simulink model "SimulationBlockDiagram"  (R2019b)
settings: Solver=VariableStepAuto  StartTime=0.0  StopTime=10.0  RelTol=1e-3
libraries: mobileRoboticsLib x3, simulink x2
settings Model: Creator=Douglas.C  LastModifiedBy=Douglas.C

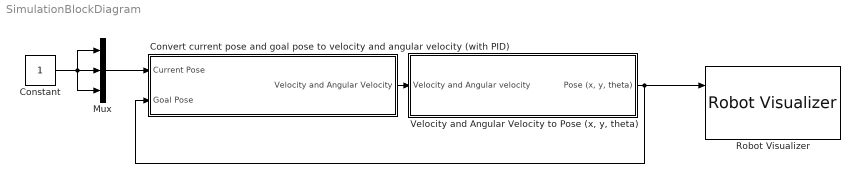
== system SimulationBlockDiagram ==
  Constant : Constant
  Convert current pose and goal pose to velocity and angular velocity (with PID) : Subsystem
  Mux : Mux  Inputs=3
  Robot Visualizer : mobileRoboticsLib/Environments/Robot Visualizer  robotRadius=0  showTrajectory=on  hasWaypoints=off  hasLidar=off  sensorOffset=[ 0, 0 ]  scanAngles=[ -pi/4, 0, pi/4 ]  hasObjDetector=on  objDetectorOffset=[ 0, 0 ]  objDetectorAngle=0  objDetectorFOV=pi/4  objDetectorMaxRange=5  objectColors=[ 1, 0, 0; 0, 1, 0; 0, 0, 1 ]  objectMarkers=s
  "Velocity and Angular Velocity to Pose (x, y, theta)" : Subsystem
  wires:
  Convert current pose and goal pose to velocity and angular velocity (with PID)/1(Velocity and Angular Velocity) -> "Velocity and Angular Velocity to Pose (x, y, theta)"/1(Velocity and Angular velocity)
  "Velocity and Angular Velocity to Pose (x, y, theta)"/1("Pose (x, y, theta)") -> Robot Visualizer/1, Convert current pose and goal pose to velocity and angular velocity (with PID)/2(Goal Pose)
  Mux/1 -> Convert current pose and goal pose to velocity and angular velocity (with PID)/1(Current Pose)
  Constant/1 -> Mux/1, Mux/3, Mux/2

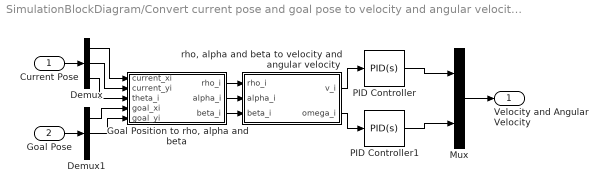
== system SimulationBlockDiagram/Convert current pose and goal pose to velocity and angular velocity (with PID) ==
  Current Pose : Inport
  Goal Pose : Inport  Port=2
  Demux : Demux  Outputs=3
  Demux1 : Demux  Outputs=3
  "Goal Position to rho, alpha and beta" : MATLAB Function  TreatAsAtomicUnit=on
  Mux : Mux  Inputs=2
  PID Controller : simulink/Continuous/PID Controller  Controller=PID  Form=Parallel  TimeDomain=Continuous-time  SampleTime=-1  IntegratorMethod=Forward Euler  FilterMethod=Forward Euler  ControllerParametersSource=internal  P=1  I=1  D=0  UseFilter=on  N=100  TunerSelectOption=Transfer Function Based (PID Tuner App)  InitialConditionSource=internal  InitialConditionForIntegrator=0  InitialConditionForFilter=0  DifferentiatorICPrevScaledInput=0  ExternalReset=none  TrackingMode=off  Kt=1  LimitOutput=off  UpperSaturationLimit=inf  LowerSaturationLimit=-inf  LinearizeAsGain=on  AntiWindupMode=none  Kb=1  POutMin=[]  POutMax=[]  IOutMin=[]  IOutMax=[]  DOutMin=[]  DOutMax=[]  NOutMin=[]  NOutMax=[]  SumOutMin=[]  SumOutMax=[]  SaturationOutMin=[]  SaturationOutMax=[]  PParamMin=[]  PParamMax=[]  IParamMin=[]  IParamMax=[]  DParamMin=[]  DParamMax=[]  NParamMin=[]  NParamMax=[]  KbParamMin=[]  KbParamMax=[]  KtParamMin=[]  KtParamMax=[]  KbOutMin=[]  KbOutMax=[]  KtOutMin=[]  KtOutMax=[]  IntegratorOutMin=[]  IntegratorOutMax=[]  FilterOutMin=[]  FilterOutMax=[]  SumI1OutMin=[]  SumI1OutMax=[]  SumI2OutMin=[]  SumI2OutMax=[]  SumI3OutMin=[]  SumI3OutMax=[]  SumI4OutMin=[]  SumI4OutMax=[]  SumDOutMin=[]  SumDOutMax=[]  DifferentiatorOutMin=[]  DifferentiatorOutMax=[]  FilterDiffOutCoefMin=[]  FilterDiffOutCoefMax=[]  ReciprocalOutMin=[]  ReciprocalOutMax=[]  SumDenOutMin=[]  SumDenOutMax=[]  SumNumOutMin=[]  SumNumOutMax=[]  DivideOutMin=[]  DivideOutMax=[]  IntegratorContinuousStateAttributes=''  IntegratorStateMustResolveToSignalObject=off  IntegratorRTWStateStorageClass=Auto  FilterContinuousStateAttributes=''  FilterStateMustResolveToSignalObject=off  FilterRTWStateStorageClass=Auto  ParallelPVariant=InternalParameters  IdealPVariant=Disabled  IVariant=InternalParameters  DVariant=InternalParameters  IntegratorVariant=Continuous  SatVariant=Disabled  AWVariant=Passthrough  PCopyVariant=Disabled  TRVariant=Disabled  FdbkBlocksVariant=Forward  IdealPFdbkVariant=Disabled  SatFdbkVariant=Disabled  DerivativeFilterVariant=ContFilter  NVariant=InternalParameters  NCopyVariant=Disabled  FilterICVariant=InternalICsFilter  IntegratorICVariant=InternalICs  ExternalResetVariant=Disabled  TRSumVariant=Passthrough  SumFdbkVariant=Disabled  SumVariant=Sum_PID
  PID Controller1 : simulink/Continuous/PID Controller  Controller=PID  Form=Parallel  TimeDomain=Continuous-time  SampleTime=-1  IntegratorMethod=Forward Euler  FilterMethod=Forward Euler  ControllerParametersSource=internal  P=1  I=1  D=0  UseFilter=on  N=100  TunerSelectOption=Transfer Function Based (PID Tuner App)  InitialConditionSource=internal  InitialConditionForIntegrator=0  InitialConditionForFilter=0  DifferentiatorICPrevScaledInput=0  ExternalReset=none  TrackingMode=off  Kt=1  LimitOutput=off  UpperSaturationLimit=inf  LowerSaturationLimit=-inf  LinearizeAsGain=on  AntiWindupMode=none  Kb=1  POutMin=[]  POutMax=[]  IOutMin=[]  IOutMax=[]  DOutMin=[]  DOutMax=[]  NOutMin=[]  NOutMax=[]  SumOutMin=[]  SumOutMax=[]  SaturationOutMin=[]  SaturationOutMax=[]  PParamMin=[]  PParamMax=[]  IParamMin=[]  IParamMax=[]  DParamMin=[]  DParamMax=[]  NParamMin=[]  NParamMax=[]  KbParamMin=[]  KbParamMax=[]  KtParamMin=[]  KtParamMax=[]  KbOutMin=[]  KbOutMax=[]  KtOutMin=[]  KtOutMax=[]  IntegratorOutMin=[]  IntegratorOutMax=[]  FilterOutMin=[]  FilterOutMax=[]  SumI1OutMin=[]  SumI1OutMax=[]  SumI2OutMin=[]  SumI2OutMax=[]  SumI3OutMin=[]  SumI3OutMax=[]  SumI4OutMin=[]  SumI4OutMax=[]  SumDOutMin=[]  SumDOutMax=[]  DifferentiatorOutMin=[]  DifferentiatorOutMax=[]  FilterDiffOutCoefMin=[]  FilterDiffOutCoefMax=[]  ReciprocalOutMin=[]  ReciprocalOutMax=[]  SumDenOutMin=[]  SumDenOutMax=[]  SumNumOutMin=[]  SumNumOutMax=[]  DivideOutMin=[]  DivideOutMax=[]  IntegratorContinuousStateAttributes=''  IntegratorStateMustResolveToSignalObject=off  IntegratorRTWStateStorageClass=Auto  FilterContinuousStateAttributes=''  FilterStateMustResolveToSignalObject=off  FilterRTWStateStorageClass=Auto  ParallelPVariant=InternalParameters  IdealPVariant=Disabled  IVariant=InternalParameters  DVariant=InternalParameters  IntegratorVariant=Continuous  SatVariant=Disabled  AWVariant=Passthrough  PCopyVariant=Disabled  TRVariant=Disabled  FdbkBlocksVariant=Forward  IdealPFdbkVariant=Disabled  SatFdbkVariant=Disabled  DerivativeFilterVariant=ContFilter  NVariant=InternalParameters  NCopyVariant=Disabled  FilterICVariant=InternalICsFilter  IntegratorICVariant=InternalICs  ExternalResetVariant=Disabled  TRSumVariant=Passthrough  SumFdbkVariant=Disabled  SumVariant=Sum_PID
  "rho, alpha and beta to velocity and angular velocity" : MATLAB Function  TreatAsAtomicUnit=on
  Velocity and Angular Velocity : Outport
  wires:
  Demux1/1 -> "Goal Position to rho, alpha and beta"/4(goal_xi)
  Goal Pose/1 -> Demux1/1
  PID Controller/1 -> Mux/1
  "rho, alpha and beta to velocity and angular velocity"/1(v_i) -> PID Controller/1
  Demux/2 -> "Goal Position to rho, alpha and beta"/2(current_yi)
  Demux1/2 -> "Goal Position to rho, alpha and beta"/5(goal_yi)
  "Goal Position to rho, alpha and beta"/2(alpha_i) -> "rho, alpha and beta to velocity and angular velocity"/2(alpha_i)
  "rho, alpha and beta to velocity and angular velocity"/2(omega_i) -> PID Controller1/1
  Demux/3 -> "Goal Position to rho, alpha and beta"/3(theta_i)
  Demux/1 -> "Goal Position to rho, alpha and beta"/1(current_xi)
  "Goal Position to rho, alpha and beta"/1(rho_i) -> "rho, alpha and beta to velocity and angular velocity"/1(rho_i)
  "Goal Position to rho, alpha and beta"/3(beta_i) -> "rho, alpha and beta to velocity and angular velocity"/3(beta_i)
  PID Controller1/1 -> Mux/2
  Current Pose/1 -> Demux/1
  Mux/1 -> Velocity and Angular Velocity/1

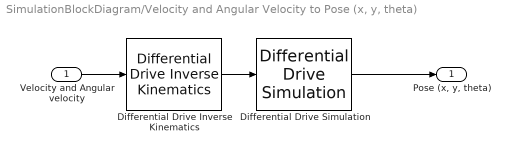
== system SimulationBlockDiagram/Velocity and Angular Velocity to Pose (x, y, theta) ==
  Velocity and Angular velocity : Inport
  Differential Drive Inverse Kinematics : mobileRoboticsLib/Kinematic Models/Differential Drive/Differential Drive Inverse Kinematics  wheelRadius=0.1  wheelBase=0.5
      settings: SourceProductName=Mobile Robotics Simulation Toolbox
  Differential Drive Simulation : mobileRoboticsLib/Kinematic Models/Differential Drive/Differential Drive Simulation  wheelRadius=0.1  wheelBase=0.5  initX=0  initY=0  initAngle=0  Ts=0.05
      settings: SourceProductName=Mobile Robotics Simulation Toolbox
  "Pose (x, y, theta)" : Outport
  wires:
  Differential Drive Simulation/1 -> "Pose (x, y, theta)"/1
  Differential Drive Inverse Kinematics/1 -> Differential Drive Simulation/1
  Velocity and Angular velocity/1 -> Differential Drive Inverse Kinematics/1

== matlab function SimulationBlockDiagram/Convert current pose and goal pose to velocity and angular velocity (with PID)/Goal Position to rho, alpha and beta ==
  data: current_xi input; rho_i output; current_yi input; alpha_i output; theta_i input; goal_xi input; goal_yi input; beta_i output
% **Description:
% This function convert the current pose and goal pose information to rho,
% alpha and beta for each robot agent
%
% **Variables Description:
%   Input:
%       current_xi: x-coordinate of current pose
%       current_yi: y-coordinate of current pose
%       theta_i:    Orientation (angle) of current pose
%
%       goal_xi:    x-coordinate of goal pose
%       goal_yi:    y-coordinate of goal pose
%
%   Output:
%       rho_i:      Distance between the Start pose and Goal pose
%       alpha_i:    Starting orientation (angle)
%       beta_i:     Goal orientation (angle)

function [rho_i, alpha_i, beta_i] = fcn(current_xi, current_yi, theta_i, goal_xi, goal_yi)
% Initialize:
rho_i    = 0.0;
alpha_i  = 0.0;
beta_i   = 0.0;

% Convert Parameters:
delta_xi = goal_xi - current_xi;
delta_yi = goal_yi - current_yi;

% Output:
rho_i    = sqrt(square(delta_xi) + square(delta_yi));
alpha_i  = atan(delta_yi/delta_xi) - theta_i;
beta_i   = - theta_i - alpha_i;

== matlab function SimulationBlockDiagram/Convert current pose and goal pose to velocity and angular velocity (with PID)/rho, alpha and beta to velocity and angular velocity ==
  data: rho_i input; v_i output; alpha_i input; omega_i output; beta_i input
% **Description:
% This function convert the information of the start pose and goal pose
% to velocity and angular velocity.
%
% **Variables Description:
%   Input:
%       rho_i:      Distance between the Start pose and Goal pose
%       alpha_i:    Starting orientation (angle)
%       beta_i:     Goal orientation (angle)
%
%   Tunning Parameters:
%       K_rho:      > 0
%       K_alpha:    > K_rho
%       K_beta:     < 0
%
%   Output:
%       v_i:        Linear velocity of robot agent i
%       omega_i:    Angular velocity of robot agent i

function [v_i, omega_i] = fcn(rho_i, alpha_i, beta_i)

% Tunning Parameters:
K_rho   = 5;
K_alpha = 10;
K_beta  = -0.1;

% Output
v_i     = K_rho*rho_i;
omega_i = K_alpha*alpha_i + K_beta*beta_i;
